simulink subsystem "subrMap"  (R2024a)
settings: Solver=VariableStepAuto  StartTime=0.0  StopTime=10.0  RelTol=1e-3
model mask{XL=1, XU=-1, YL=1, YU=0}
  mask prompts: XL "Input Lower Limit"; XU "Input Upper Limit"; YL "Output Lower Limit"; YU "Output Upper Limit"
settings Model: Creator=anant  LastModifiedBy=anant

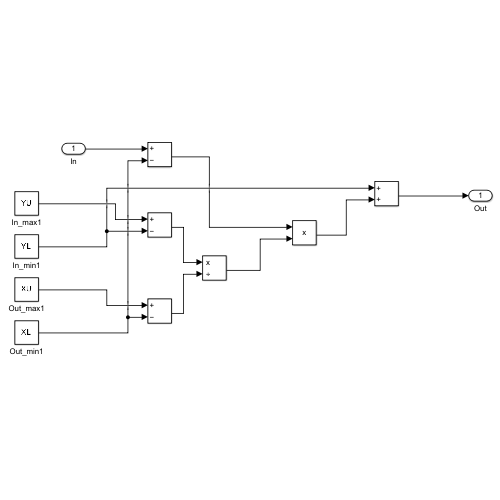
[thumbnail: Simulink's stored preview of the top-level diagram]
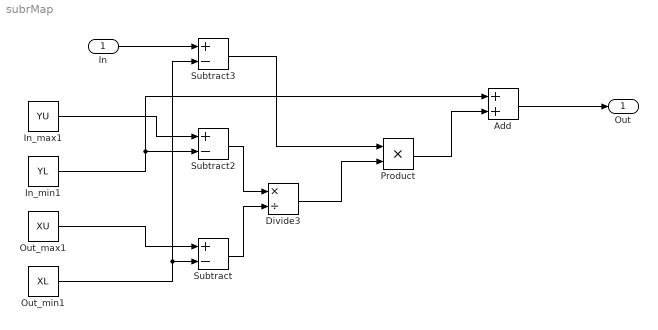
== system subrMap ==
  In : Inport
  Add : Sum
  Divide3 : Product  Inputs=*/
  In_max1 : Constant  Value=YU
  In_min1 : Constant  Value=YL
  Out_max1 : Constant  Value=XU
  Out_min1 : Constant  Value=XL
  Product : Product
  Subtract : Sum  Inputs=+-
  Subtract2 : Sum  Inputs=+-
  Subtract3 : Sum  Inputs=+-
  Out : Outport
  wires:
  Out_max1/1 -> Subtract/1
  Product/1 -> Add/2
  Subtract3/1 -> Product/1
  Subtract2/1 -> Divide3/1
  Divide3/1 -> Product/2
  Subtract/1 -> Divide3/2
  In_max1/1 -> Subtract2/1
  Out_min1/1 -> Subtract/2, Subtract3/2
  Add/1 -> Out/1
  In/1 -> Subtract3/1
  In_min1/1 -> Subtract2/2, Add/1
